simulink model "Car1"  (R2024a)
settings: Solver=VariableStepAuto  StartTime=0.0  StopTime=10.0  RelTol=1e-3
libraries: arduinolib x7
settings Model: Creator=thipp  LastModifiedBy=thipp

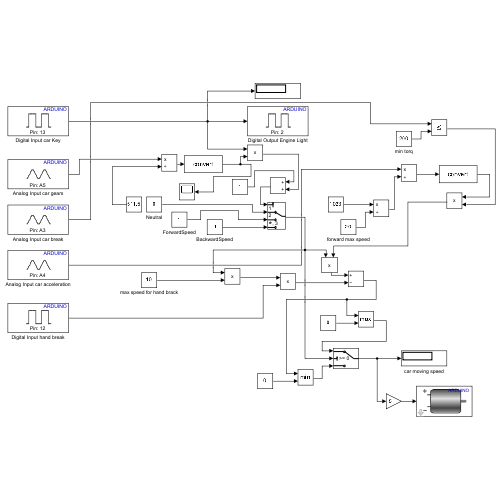
[thumbnail: Simulink's stored preview of the top-level diagram]
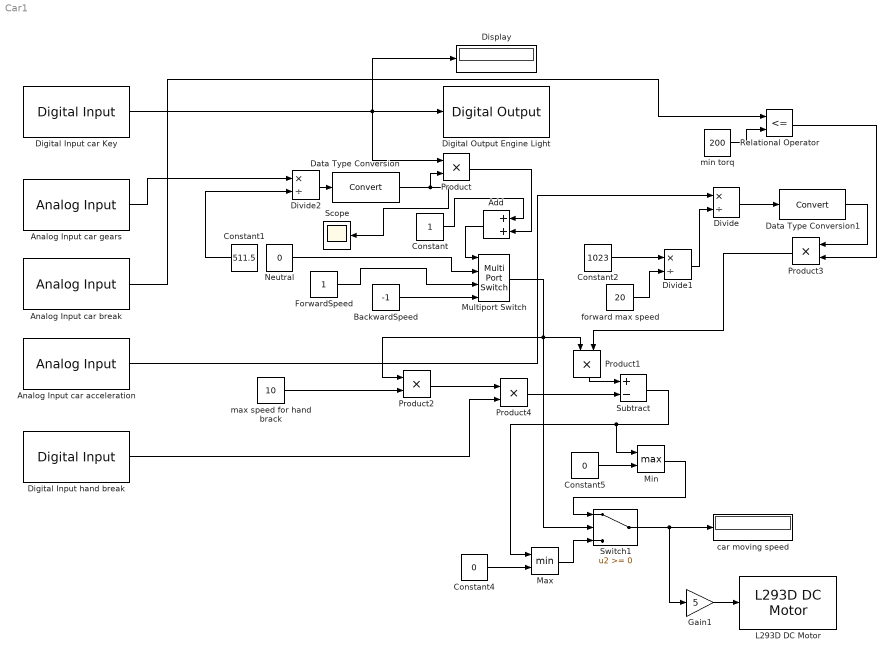
== system Car1 ==
  Add : Sum
  Analog Input car acceleration : arduinolib/Analog Input  pinNumber=4  ReadResultsOnly=off  ConversionTriggerSource=Software  ExternalTriggerType=uint32( 0 )  OutputDataType=uint16  EnableConversionCompleteNotify=off  EnableOuputStatus=off  SampleTime=-1  blockPlatform=arduino
  Analog Input car break : arduinolib/Analog Input  pinNumber=3  ReadResultsOnly=off  ConversionTriggerSource=Software  ExternalTriggerType=uint32( 0 )  OutputDataType=uint16  EnableConversionCompleteNotify=off  EnableOuputStatus=off  SampleTime=-1  blockPlatform=arduino
  Analog Input car gears : arduinolib/Analog Input  pinNumber=5  ReadResultsOnly=off  ConversionTriggerSource=Software  ExternalTriggerType=uint32( 0 )  OutputDataType=uint16  EnableConversionCompleteNotify=off  EnableOuputStatus=off  SampleTime=-1  blockPlatform=arduino
  BackwardSpeed : Constant  Value=-1
  Constant : Constant
  Constant1 : Constant  Value=511.5
  Constant2 : Constant  Value=1023
  Constant4 : Constant  Value=0
  Constant5 : Constant  Value=0
  Data Type Conversion : DataTypeConversion  SaturateOnIntegerOverflow=off  RndMeth=Floor
  Data Type Conversion1 : DataTypeConversion  SaturateOnIntegerOverflow=off  RndMeth=Floor
  Digital Input car Key : arduinolib/Digital Input  pinNumber=13  mode=Default  Direction=input  SampleTime=0.1  blockPlatform=arduino
  Digital Input hand break : arduinolib/Digital Input  pinNumber=12  mode=Default  Direction=input  SampleTime=0.1  blockPlatform=arduino
  Digital Output Engine Light : arduinolib/Digital Output  pinNumber=2  Direction=output  blockPlatform=arduino
  Display : Display
  Divide : Product  Inputs=*/  RndMeth=Zero  SaturateOnIntegerOverflow=on
  Divide1 : Product  Inputs=*/  RndMeth=Zero  SaturateOnIntegerOverflow=on
  Divide2 : Product  Inputs=*/  RndMeth=Zero  SaturateOnIntegerOverflow=on
  ForwardSpeed : Constant
  Gain1 : Gain  Gain=5
  L293D DC Motor : arduinolib/L293D DC Motor  EnablePin=11  InputAPin=10  InputBPin=9
  Max : MinMax  Inputs=2
  Min : MinMax  Function=max  Inputs=2
  Multiport Switch : MultiPortSwitch  SaturateOnIntegerOverflow=off  InputSameDT=off
  Neutral : Constant  Value=0
  Product{,1..4} (5 alike) : Product
  Relational Operator : RelationalOperator  Operator=<=  OutDataTypeStr=boolean  RndMeth=Simplest  InputSameDT=off
  Scope : Scope
  Subtract : Sum  Inputs=+-
  Switch1 : Switch  SaturateOnIntegerOverflow=off  InputSameDT=off
  car moving speed : Display
  forward max speed : Constant  Value=20
  max speed for hand brack : Constant  Value=10
  min torq : Constant  Value=200
  wires:
  BackwardSpeed/1 -> Multiport Switch/4
  Neutral/1 -> Multiport Switch/2
  ForwardSpeed/1 -> Multiport Switch/3
  Analog Input car gears/1 -> Divide2/1
  Multiport Switch/1 -> Product2/1, Product1/1, Switch1/2
  Analog Input car acceleration/1 -> Divide/1
  Divide1/1 -> Divide/2
  Constant2/1 -> Divide1/1
  forward max speed/1 -> Divide1/2
  Divide/1 -> Data Type Conversion1/1
  max speed for hand brack/1 -> Product2/2
  Product1/1 -> Subtract/1
  Product2/1 -> Product4/1
  Digital Input hand break/1 -> Product4/2
  Product4/1 -> Subtract/2
  Min/1 -> Switch1/1
  Constant5/1 -> Min/2
  Subtract/1 -> Min/1, Max/1
  Constant4/1 -> Max/2
  Max/1 -> Switch1/3
  Switch1/1 -> Gain1/1, car moving speed/1
  Analog Input car break/1 -> Relational Operator/1
  min torq/1 -> Relational Operator/2
  Data Type Conversion1/1 -> Product3/1
  Relational Operator/1 -> Product3/2
  Product3/1 -> Product1/2
  Gain1/1 -> L293D DC Motor/1
  Product/1 -> Add/2
  Add/1 -> Multiport Switch/1
  Constant/1 -> Add/1
  Divide2/1 -> Data Type Conversion/1
  Data Type Conversion/1 -> Scope/1, Product/2
  Constant1/1 -> Divide2/2
  Digital Input car Key/1 -> Display/1, Digital Output Engine Light/1, Product/1
